simulink model "hw1"  (R2022a)
settings: Solver=VariableStepAuto  StartTime=0.0  StopTime=10.0  RelTol=1e-3
settings Model: Creator=Ariike.ir  LastModifiedBy=Ariike.ir

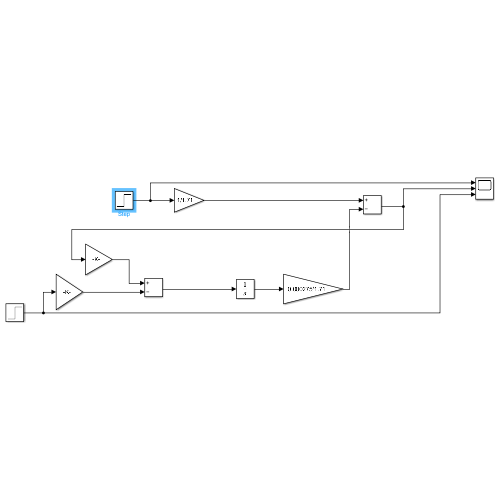
[thumbnail: Simulink's stored preview of the top-level diagram]
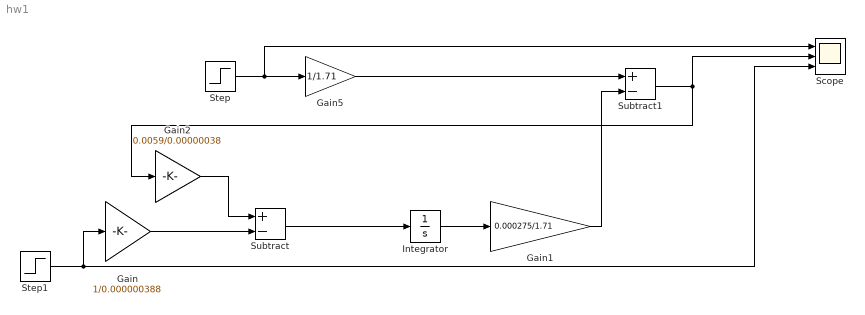
== system hw1 ==
  Gain : Gain  Gain=1/0.000000388
  Gain1 : Gain  Gain=0.000275/1.71
  Gain2 : Gain  Gain=0.0059/0.00000038
  Gain5 : Gain  Gain=1/1.71
  Integrator : Integrator
  Scope : Scope  NumInputPorts=3
  Step : Step  Time=5  After=5  SampleTime=0
  Step1 : Step  Time=5  After=0.01  SampleTime=0
  Subtract : Sum  Inputs=+-
  Subtract1 : Sum  Inputs=+-
  wires:
  Gain1/1 -> Subtract1/2
  Gain/1 -> Subtract/2
  Gain2/1 -> Subtract/1
  Step1/1 -> Scope/3, Gain/1
  Subtract/1 -> Integrator/1
  Integrator/1 -> Gain1/1
  Step/1 -> Scope/1, Gain5/1
  Gain5/1 -> Subtract1/1
  Subtract1/1 -> Gain2/1, Scope/2
